simulink model "exampleWeatherFromFile"  (R2016b)
settings: Solver=ode45  StartTime=90*24*3600  StopTime=100*24*3600  RelTol=1e-3  EnableMultiTasking=on
libraries: carnot x1
settings Model: Creator=drhf  LastModifiedBy=drhf
settings DataIOCC: LimitDataPoints=on  SaveFormat=Array  SignalLoggingSaveFormat=ModelDataLogs
settings OptimizationCC: ExpressionDepthLimit=2147483647  LifeSpan=inf
settings DebuggingCC: UnderspecifiedInitializationDetection=Classic  MergeDetectMultiDrivingBlocksExec=none  SolverPrmCheckMsg=warning  StateNameClashWarn=warning  SFUnexpectedBacktrackingDiag=warning  SFNoUnconditionalDefaultTransitionDiag=warning  SFExecutionAtInitializationDiag=none
settings HardwareCC: ProdBitPerPointer=32  ProdBitPerSizeT=32  ProdBitPerPtrDiffT=32  ProdLargestAtomicFloat=None  ProdIntDivRoundTo=Undefined  ProdEndianess=Unspecified  ProdWordSize=32  ProdHWDeviceType=32-bit Generic
settings ModelReferenceCC: PropagateSignalLabelsOutOfModel=off
settings GRTTargetCC: TargetLangStandard=C89/C90 (ANSI)  GeneratePreprocessorConditionals=Disable all  CombineOutputUpdateFcns=off  GRTInterface=on
settings ConfigComp: CovMetricSettings=dw  CovHtmlReporting=on  CovSaveCumulativeToWorkspaceVar=on  CovSaveSingleToWorkspaceVar=on  CovExternalEMLEnable=off

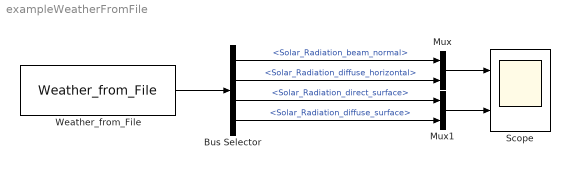
== system exampleWeatherFromFile ==
  Bus Selector : BusSelector  OutputSignals=Solar_Radiation_beam_normal,Solar_Radiation_diffuse_horizontal,Solar_Radiation_direct_surface,Solar_Radiation_diffuse_surface
  Mux : Mux  Inputs=2
  Mux1 : Mux  Inputs=2
  Scope : Scope  NumInputPorts=2
  Weather_from_File : carnot/Weather/Weather_from_File  file=DE_TRY2010_08_averageYear  ext=.mat
  wires:
  Weather_from_File/1 -> Bus Selector/1
  Bus Selector/1 -> Mux/1  "<Solar_Radiation_beam_normal>"
  Bus Selector/2 -> Mux/2  "<Solar_Radiation_diffuse_horizontal>"
  Bus Selector/3 -> Mux1/1  "<Solar_Radiation_direct_surface>"
  Bus Selector/4 -> Mux1/2  "<Solar_Radiation_diffuse_surface>"
  Mux/1 -> Scope/1
  Mux1/1 -> Scope/2
